simulink model "drone_level_2"  (R2023a)
settings: Solver=VariableStepAuto  StartTime=0.0  StopTime=10.0  RelTol=1e-3
values from neighbouring files (symbols this model uses):
  Kp_omega = 10    [tuning.m]
undefined symbols (not defined in the file or in its folder): dxdt
libraries: simulink x1
settings Model: Creator=timme  LastModifiedBy=timme
settings OptimizationCC: BlockReduction=off  DefaultParameterBehavior=Inlined  BufferReuse=off

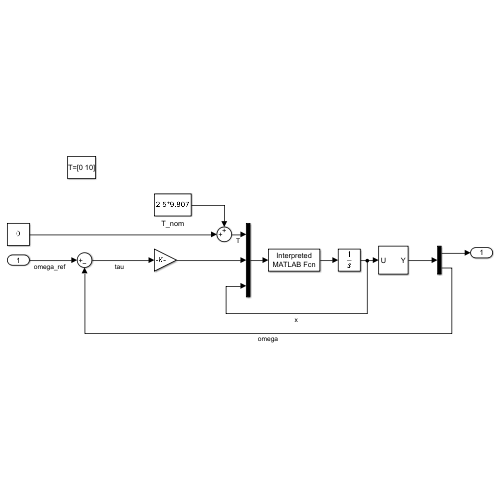
[thumbnail: Simulink's stored preview of the top-level diagram]
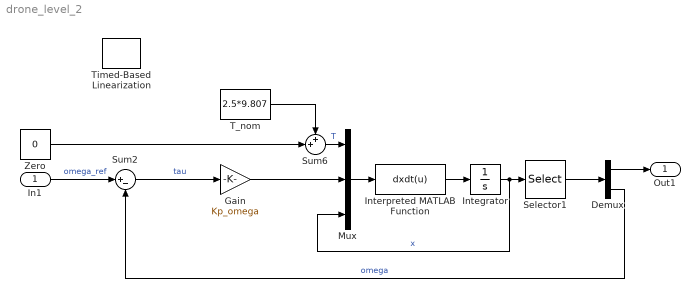
== system drone_level_2 ==
  In1 : Inport
  Demux : Demux  Outputs=2
  Gain : Gain  Gain=Kp_omega
  Integrator : Integrator  InitialCondition=zeros(6,1)
  Interpreted MATLAB Function : MATLABFcn  MATLABFcn=dxdt(u)  OutputDimensions=6
  Mux : Mux  Inputs=3
  Selector1 : Selector  InputPortWidth=6  IndexOptions=Index vector (dialog)  Indices=[3, 6]  OutputSizes=1
  Sum2 : Sum  Inputs=|+-
  Sum6 : Sum  Inputs=++|
  T_nom : Constant  Value=2.5*9.807
  Timed-Based Linearization : simulink/Model-Wide Utilities/Timed-Based Linearization  LinearizationTime=[0 10]  SampleTime=0
  Zero : Constant  Value=0  OutDataTypeStr=Inherit: Inherit via back propagation
  Out1 : Outport
  wires:
  Sum2/1 -> Gain/1  "tau"
  Zero/1 -> Sum6/2
  Selector1/1 -> Demux/1
  Mux/1 -> Interpreted MATLAB Function/1
  Interpreted MATLAB Function/1 -> Integrator/1
  Sum6/1 -> Mux/1  "T"
  Integrator/1 -> Selector1/1, Mux/3  "x"
  T_nom/1 -> Sum6/1
  In1/1 -> Sum2/1  "omega_ref"
  Demux/2 -> Sum2/2  "omega"
  Demux/1 -> Out1/1
  Gain/1 -> Mux/2
